simulink model "SimpleVehicle"  (R2018b)
settings: Solver=FixedStepAuto  StartTime=0.0  StopTime=stop_time  FixedStep=global_time_step  RelTol=1e-3
undefined symbols (not defined in the file): car_mass, driver_mass
libraries: nesl_utility x22, fl_lib x12, sdl_lib x5
settings Model: Creator=jbray  LastModifiedBy=Dylan

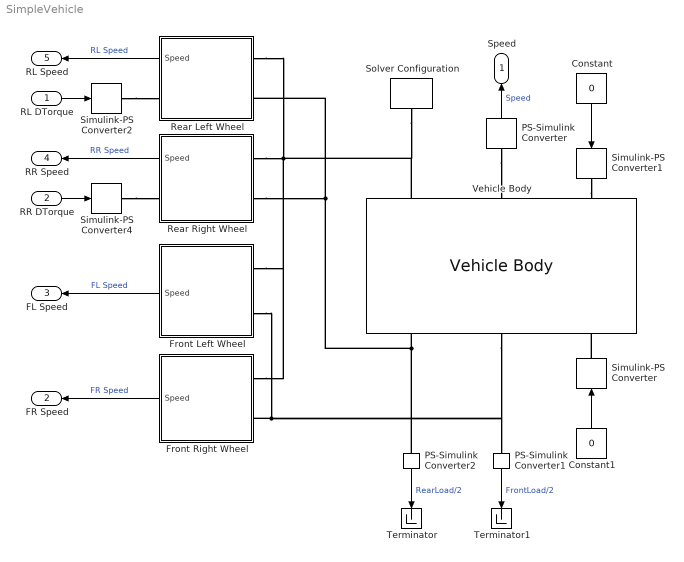
== system SimpleVehicle ==
  RL DTorque : Inport
  RR DTorque : Inport  Port=2
  Constant : Constant  Value=0
  Constant1 : Constant  Value=0
  Front Left Wheel : Subsystem
  Front Right Wheel : Subsystem
  PS-Simulink Converter : nesl_utility/PS-Simulink Converter  PhysicalDomain=network_engine_domain  SubClassName=ps_output  LeftPortType=input  RightPortType=output  PseudoPeriodic=off  Frequencies=[]  Unit=m/s  AffineConversion=off
  PS-Simulink Converter1 : nesl_utility/PS-Simulink Converter  PhysicalDomain=network_engine_domain  SubClassName=ps_output  LeftPortType=input  RightPortType=output  PseudoPeriodic=off  Frequencies=[]  Unit=N  AffineConversion=off
  PS-Simulink Converter2 : nesl_utility/PS-Simulink Converter  PhysicalDomain=network_engine_domain  SubClassName=ps_output  LeftPortType=input  RightPortType=output  PseudoPeriodic=off  Frequencies=[]  Unit=N  AffineConversion=off
  Rear Left Wheel : Subsystem
  Rear Right Wheel : Subsystem
  Simulink-PS Converter : nesl_utility/Simulink-PS Converter  PhysicalDomain=network_engine_domain  SubClassName=ps_input  LeftPortType=input  RightPortType=output  PseudoPeriodic=off  Frequencies=[]  NoiseDistribution=none  NoiseParameters=[]  Unit=rad  AffineConversion=off  FilteringAndDerivatives=provide  SimscapeFilterOrder=1  InputFilterTimeConstant=0.001  UdotUserProvided=0
  Simulink-PS Converter1 : nesl_utility/Simulink-PS Converter  PhysicalDomain=network_engine_domain  SubClassName=ps_input  LeftPortType=input  RightPortType=output  PseudoPeriodic=off  Frequencies=[]  NoiseDistribution=none  NoiseParameters=[]  Unit=m/s  AffineConversion=off  FilteringAndDerivatives=provide  SimscapeFilterOrder=1  InputFilterTimeConstant=0.001  UdotUserProvided=0
  Simulink-PS Converter2 : nesl_utility/Simulink-PS Converter  PhysicalDomain=network_engine_domain  SubClassName=ps_input  LeftPortType=input  RightPortType=output  PseudoPeriodic=off  Frequencies=[]  NoiseDistribution=none  NoiseParameters=[]  Unit=N*m  AffineConversion=off  FilteringAndDerivatives=provide  SimscapeFilterOrder=1  InputFilterTimeConstant=0.001  UdotUserProvided=0
  Simulink-PS Converter4 : nesl_utility/Simulink-PS Converter  PhysicalDomain=network_engine_domain  SubClassName=ps_input  LeftPortType=input  RightPortType=output  PseudoPeriodic=off  Frequencies=[]  NoiseDistribution=none  NoiseParameters=[]  Unit=N*m  AffineConversion=off  FilteringAndDerivatives=provide  SimscapeFilterOrder=1  InputFilterTimeConstant=0.001  UdotUserProvided=0
  Solver Configuration : nesl_utility/Solver Configuration  PhysicalDomain=network_engine_domain  SubClassName=solver  LeftPortType=input  RightPortType=generic  Tones=[]  Harmonics=[]  SimulateNoise=off  Profile=off  UseLocalSampling=off  EnableSwitchedLinearOptims=on  FrequencyDomain=off  UseCCode=off  RelTol=0.001  AbsTol=1e-06  MinStep=1e-09  ToWorkspace=off  RevertToSquareIcSolve=off  NumHomotopyIterations=100  PhasorMode=off  PhasorModeNumHarmonics=1  DoDC=off  ResidualTolerance=1e-09  UseLocalSolver=off  LocalSolverChoice=NE_BACKWARD_EULER_ADVANCER  LocalSolverSampleTime=0.001  DoFixedCost=off  MaxNonlinIter=3  MaxModeIter=2  LinearAlgebra=Sparse  EquationFormulation=NE_TIME_EF  DelaysMemoryBudget=1024  AutomaticFiltering=on  FilteringTimeConstant=0.001  PartitionStorageMethod=AS_NEEDED  PartitionMemoryBudget=1024
  Terminator : Terminator
  Terminator1 : Terminator
  Vehicle Body : sdl_lib/Tires & Vehicles/Vehicle Body  mass=car_mass+driver_mass kg  n_w=2  x_f=CG_front m  x_r=CG_rear m  y_c=CG_height m  model_pitch=1  inertia=pitch_moment_of_inertia kg*m^2  suspension_model=1  k_f=front_suspension_stiffness N/m  b_f=front_suspension_damping N/(m/s)  k_r=rear_suspension_stiffness N/m  b_r=rear_suspension_damping N/(m/s)  k_f_TLU=[-2000, -1000, 0, 1000, 2000] N  x_f_TLU=[-.4, -.2, 0, .2, .4] m  b_f_TLU=[-200, -100, 0, 100, 200] N  v_f_TLU=[-4, -2, 0, 2, 4] m/s  k_r_TLU=[-2000, -1000, 0, 1000, 2000] N  x_r_TLU=[-.4, -.2, 0, .2, .4] m  b_r_TLU=[-200, -100, 0, 100, 200] N  v_r_TLU=[-4, -2, 0, 2, 4] m/s  interp_method=simscape.enum.interpolation.linear  extrap_method=simscape.enum.extrapolation.linear  model_hardstop=0  upper_bound_f=.25 m  lower_bound_f=-.25 m  stop_k_f=1e6 N/m  stop_b_f=150 N/(m/s)  upper_bound_r=.25 m  lower_bound_r=-.25 m  stop_k_r=1e6 N/m  stop_b_r=150 N/(m/s)  initial_pitch=0 rad  initial_pitch_rate=0 rad/s  g=9.81 m/s^2  liftoff_warning=0  area=frontal_area m^2  Cd=drag_coeff  rho=air_density kg/m^3  v_specify=off  v_priority=High  v=0 m/s  v_nominal_specify=off  v_nominal_unit=m/s  v_nominal_value=1
      settings: SourceProductName=Simscape Driveline
  Speed : Outport
  FR Speed : Outport  Port=2
  FL Speed : Outport  Port=3
  RR Speed : Outport  Port=4
  RL Speed : Outport  Port=5
  wires:
  Constant/1 -> Simulink-PS Converter1/1
  RL DTorque/1 -> Simulink-PS Converter2/1
  PS-Simulink Converter/1 -> Speed/1  "Speed"
  PS-Simulink Converter1/1 -> Terminator1/1  "FrontLoad/2"
  PS-Simulink Converter2/1 -> Terminator/1  "RearLoad/2"
  Constant1/1 -> Simulink-PS Converter/1
  Front Right Wheel/1(Speed) -> FR Speed/1  "FR Speed"
  Front Left Wheel/1(Speed) -> FL Speed/1  "FL Speed"
  RR DTorque/1 -> Simulink-PS Converter4/1
  Rear Left Wheel/1(Speed) -> RL Speed/1  "RL Speed"
  Rear Right Wheel/1(Speed) -> RR Speed/1  "RR Speed"
  connections:
  Front Left Wheel/LConn2 -- Vehicle Body/RConn2 -- PS-Simulink Converter1/LConn1 -- Front Right Wheel/LConn2
  Vehicle Body/RConn1 -- PS-Simulink Converter2/LConn1 -- Rear Right Wheel/LConn2 -- Rear Left Wheel/LConn2
  Rear Right Wheel/LConn1 -- Front Left Wheel/LConn1 -- Front Right Wheel/LConn1 -- Rear Left Wheel/LConn1 -- Vehicle Body/LConn1 -- Solver Configuration/RConn1
  Simulink-PS Converter4/RConn1 -- Rear Right Wheel/RConn1
  Simulink-PS Converter2/RConn1 -- Rear Left Wheel/RConn1
  Simulink-PS Converter/RConn1 -- Vehicle Body/RConn3
  PS-Simulink Converter/LConn1 -- Vehicle Body/LConn2
  Simulink-PS Converter1/RConn1 -- Vehicle Body/LConn3

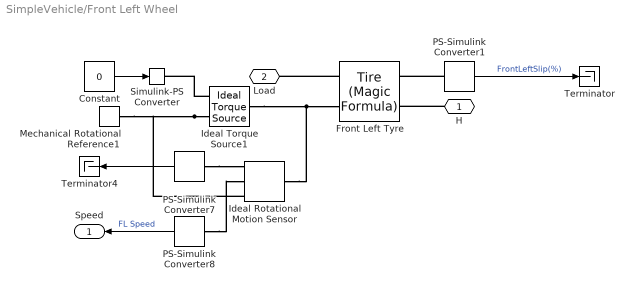
== system SimpleVehicle/Front Left Wheel ==
  Constant : Constant  Value=0
  Front Left Tyre : sdl_lib/Tires & Vehicles/Tire (Magic Formula)  parameterization=2  F_z1=3000 N  F_x1=3500 N  kappa1=10  B_m=magic_B  C_m=magic_C  D_m=magic_D  E_m=magic_E  fz0=4000 N  p_Cx=1.685  p_Dx=[1.21, -.037]  p_Ex=[.344, .095, -.02, 0]  p_Kx=[21.51, -.163, .245]  p_Hx=[-.002, .002]  p_Vx=[0, 0]  v_tr_thr=0.1 m/s  r_e=tyre_radius m  model_compliance=1  stiffness=tyre_stiffness N/m  damping=tyre_damping N/(m/s)  model_inertia=1  inertia=tyre_inertia kg*m^2  initial_velocity=0 rad/s  model_resistance=0  resistance_model=1  coeff=0.015  p_tire=250e3 Pa  alpha=-0.003  beta=0.97  coeff_a=84e-4  coeff_b=6.2e-4 s/m  coeff_c=1.6e-4 s^2/m^2  v_thr=0.001 m/s
      settings: SourceProductName=Simscape Driveline
  Ideal Rotational Motion Sensor : fl_lib/Mechanical/Mechanical Sensors/Ideal Rotational Motion Sensor  offset=0 rad
  Ideal Torque Source1 : fl_lib/Mechanical/Mechanical Sources/Ideal Torque Source
  Mechanical Rotational Reference1 : fl_lib/Mechanical/Rotational Elements/Mechanical Rotational Reference
  PS-Simulink Converter1 : nesl_utility/PS-Simulink Converter  PhysicalDomain=network_engine_domain  SubClassName=ps_output  LeftPortType=input  RightPortType=output  PseudoPeriodic=off  Frequencies=[]  Unit=1  AffineConversion=off
  PS-Simulink Converter7 : nesl_utility/PS-Simulink Converter  PhysicalDomain=network_engine_domain  SubClassName=ps_output  LeftPortType=input  RightPortType=output  PseudoPeriodic=off  Frequencies=[]  Unit=rad  AffineConversion=off
  PS-Simulink Converter8 : nesl_utility/PS-Simulink Converter  PhysicalDomain=network_engine_domain  SubClassName=ps_output  LeftPortType=input  RightPortType=output  PseudoPeriodic=off  Frequencies=[]  Unit=rad/s  AffineConversion=off
  Simulink-PS Converter : nesl_utility/Simulink-PS Converter  PhysicalDomain=network_engine_domain  SubClassName=ps_input  LeftPortType=input  RightPortType=output  PseudoPeriodic=off  Frequencies=[]  NoiseDistribution=none  NoiseParameters=[]  Unit=1  AffineConversion=off  FilteringAndDerivatives=provide  SimscapeFilterOrder=1  InputFilterTimeConstant=0.001  UdotUserProvided=0
  Terminator : Terminator
  Terminator4 : Terminator
  H : PMIOPort  Side=Left
  Load : PMIOPort  Port=2  Side=Left
  Speed : Outport
  wires:
  PS-Simulink Converter1/1 -> Terminator/1  "FrontLeftSlip(%)"
  PS-Simulink Converter8/1 -> Speed/1  "FL Speed"
  PS-Simulink Converter7/1 -> Terminator4/1
  Constant/1 -> Simulink-PS Converter/1
  connections:
  Front Left Tyre/LConn1 -- Load/RConn1
  PS-Simulink Converter1/LConn1 -- Front Left Tyre/RConn1
  H/RConn1 -- Front Left Tyre/RConn2
  PS-Simulink Converter7/LConn1 -- Ideal Rotational Motion Sensor/RConn3
  PS-Simulink Converter8/LConn1 -- Ideal Rotational Motion Sensor/RConn2
  Ideal Torque Source1/RConn1 -- Simulink-PS Converter/RConn1
  Ideal Rotational Motion Sensor/LConn1 -- Ideal Torque Source1/LConn1 -- Front Left Tyre/LConn2
  Ideal Torque Source1/RConn2 -- Ideal Rotational Motion Sensor/RConn1 -- Mechanical Rotational Reference1/LConn1

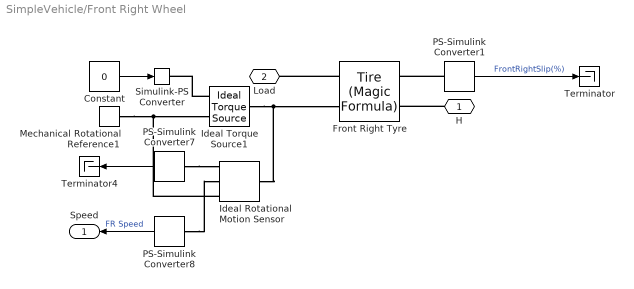
== system SimpleVehicle/Front Right Wheel ==
  Constant : Constant  Value=0
  Front Right Tyre : sdl_lib/Tires & Vehicles/Tire (Magic Formula)  parameterization=2  F_z1=3000 N  F_x1=3500 N  kappa1=10  B_m=magic_B  C_m=magic_C  D_m=magic_D  E_m=magic_E  fz0=4000 N  p_Cx=1.685  p_Dx=[1.21, -.037]  p_Ex=[.344, .095, -.02, 0]  p_Kx=[21.51, -.163, .245]  p_Hx=[-.002, .002]  p_Vx=[0, 0]  v_tr_thr=0.1 m/s  r_e=tyre_radius m  model_compliance=1  stiffness=tyre_stiffness N/m  damping=tyre_damping N/(m/s)  model_inertia=1  inertia=tyre_inertia kg*m^2  initial_velocity=0 rad/s  model_resistance=0  resistance_model=1  coeff=0.015  p_tire=250e3 Pa  alpha=-0.003  beta=0.97  coeff_a=84e-4  coeff_b=6.2e-4 s/m  coeff_c=1.6e-4 s^2/m^2  v_thr=0.001 m/s
      settings: SourceProductName=Simscape Driveline
  Ideal Rotational Motion Sensor : fl_lib/Mechanical/Mechanical Sensors/Ideal Rotational Motion Sensor  offset=0 rad
  Ideal Torque Source1 : fl_lib/Mechanical/Mechanical Sources/Ideal Torque Source
  Mechanical Rotational Reference1 : fl_lib/Mechanical/Rotational Elements/Mechanical Rotational Reference
  PS-Simulink Converter1 : nesl_utility/PS-Simulink Converter  PhysicalDomain=network_engine_domain  SubClassName=ps_output  LeftPortType=input  RightPortType=output  PseudoPeriodic=off  Frequencies=[]  Unit=1  AffineConversion=off
  PS-Simulink Converter7 : nesl_utility/PS-Simulink Converter  PhysicalDomain=network_engine_domain  SubClassName=ps_output  LeftPortType=input  RightPortType=output  PseudoPeriodic=off  Frequencies=[]  Unit=rad  AffineConversion=off
  PS-Simulink Converter8 : nesl_utility/PS-Simulink Converter  PhysicalDomain=network_engine_domain  SubClassName=ps_output  LeftPortType=input  RightPortType=output  PseudoPeriodic=off  Frequencies=[]  Unit=rad/s  AffineConversion=off
  Simulink-PS Converter : nesl_utility/Simulink-PS Converter  PhysicalDomain=network_engine_domain  SubClassName=ps_input  LeftPortType=input  RightPortType=output  PseudoPeriodic=off  Frequencies=[]  NoiseDistribution=none  NoiseParameters=[]  Unit=1  AffineConversion=off  FilteringAndDerivatives=provide  SimscapeFilterOrder=1  InputFilterTimeConstant=0.001  UdotUserProvided=0
  Terminator : Terminator
  Terminator4 : Terminator
  H : PMIOPort  Side=Left
  Load : PMIOPort  Port=2  Side=Left
  Speed : Outport
  wires:
  PS-Simulink Converter7/1 -> Terminator4/1
  PS-Simulink Converter8/1 -> Speed/1  "FR Speed"
  PS-Simulink Converter1/1 -> Terminator/1  "FrontRightSlip(%)"
  Constant/1 -> Simulink-PS Converter/1
  connections:
  Mechanical Rotational Reference1/LConn1 -- Ideal Torque Source1/RConn2 -- Ideal Rotational Motion Sensor/RConn1
  Ideal Torque Source1/LConn1 -- Front Right Tyre/LConn2 -- Ideal Rotational Motion Sensor/LConn1
  Ideal Torque Source1/RConn1 -- Simulink-PS Converter/RConn1
  PS-Simulink Converter8/LConn1 -- Ideal Rotational Motion Sensor/RConn2
  PS-Simulink Converter7/LConn1 -- Ideal Rotational Motion Sensor/RConn3
  H/RConn1 -- Front Right Tyre/RConn2
  PS-Simulink Converter1/LConn1 -- Front Right Tyre/RConn1
  Front Right Tyre/LConn1 -- Load/RConn1

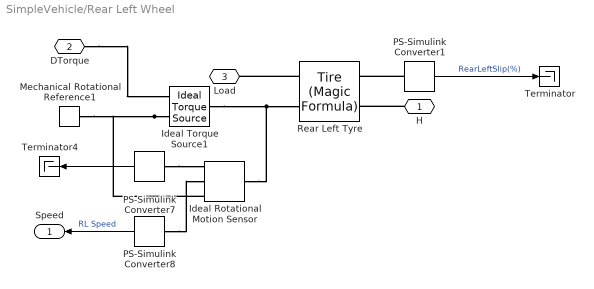
== system SimpleVehicle/Rear Left Wheel ==
  Ideal Rotational Motion Sensor : fl_lib/Mechanical/Mechanical Sensors/Ideal Rotational Motion Sensor  offset=0 rad
  Ideal Torque Source1 : fl_lib/Mechanical/Mechanical Sources/Ideal Torque Source
  Mechanical Rotational Reference1 : fl_lib/Mechanical/Rotational Elements/Mechanical Rotational Reference
  PS-Simulink Converter1 : nesl_utility/PS-Simulink Converter  PhysicalDomain=network_engine_domain  SubClassName=ps_output  LeftPortType=input  RightPortType=output  PseudoPeriodic=off  Frequencies=[]  Unit=1  AffineConversion=off
  PS-Simulink Converter7 : nesl_utility/PS-Simulink Converter  PhysicalDomain=network_engine_domain  SubClassName=ps_output  LeftPortType=input  RightPortType=output  PseudoPeriodic=off  Frequencies=[]  Unit=rad  AffineConversion=off
  PS-Simulink Converter8 : nesl_utility/PS-Simulink Converter  PhysicalDomain=network_engine_domain  SubClassName=ps_output  LeftPortType=input  RightPortType=output  PseudoPeriodic=off  Frequencies=[]  Unit=rad/s  AffineConversion=off
  Rear Left Tyre : sdl_lib/Tires & Vehicles/Tire (Magic Formula)  parameterization=2  F_z1=3000 N  F_x1=3500 N  kappa1=10  B_m=magic_B  C_m=magic_C  D_m=magic_D  E_m=magic_E  fz0=4000 N  p_Cx=1.685  p_Dx=[1.21, -.037]  p_Ex=[.344, .095, -.02, 0]  p_Kx=[21.51, -.163, .245]  p_Hx=[-.002, .002]  p_Vx=[0, 0]  v_tr_thr=0.1 m/s  r_e=tyre_radius m  model_compliance=1  stiffness=tyre_stiffness N/m  damping=tyre_damping N/(m/s)  model_inertia=1  inertia=tyre_inertia kg*m^2  initial_velocity=0 rad/s  model_resistance=0  resistance_model=1  coeff=0.015  p_tire=250e3 Pa  alpha=-0.003  beta=0.97  coeff_a=84e-4  coeff_b=6.2e-4 s/m  coeff_c=1.6e-4 s^2/m^2  v_thr=0.001 m/s
      settings: SourceProductName=Simscape Driveline
  Terminator : Terminator
  Terminator4 : Terminator
  H : PMIOPort  Side=Left
  DTorque : PMIOPort  Port=2  Side=Right
  Load : PMIOPort  Port=3  Side=Left
  Speed : Outport
  wires:
  PS-Simulink Converter1/1 -> Terminator/1  "RearLeftSlip(%)"
  PS-Simulink Converter8/1 -> Speed/1  "RL Speed"
  PS-Simulink Converter7/1 -> Terminator4/1
  connections:
  Rear Left Tyre/LConn1 -- Load/RConn1
  PS-Simulink Converter1/LConn1 -- Rear Left Tyre/RConn1
  H/RConn1 -- Rear Left Tyre/RConn2
  PS-Simulink Converter7/LConn1 -- Ideal Rotational Motion Sensor/RConn3
  PS-Simulink Converter8/LConn1 -- Ideal Rotational Motion Sensor/RConn2
  DTorque/RConn1 -- Ideal Torque Source1/RConn1
  Ideal Rotational Motion Sensor/LConn1 -- Ideal Torque Source1/LConn1 -- Rear Left Tyre/LConn2
  Ideal Torque Source1/RConn2 -- Ideal Rotational Motion Sensor/RConn1 -- Mechanical Rotational Reference1/LConn1

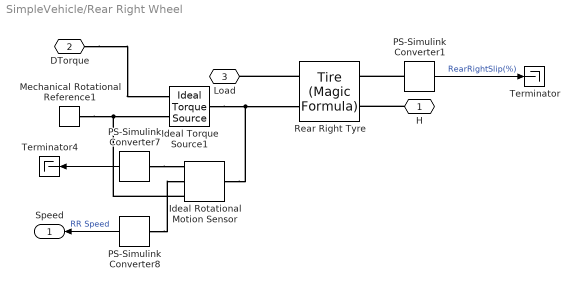
== system SimpleVehicle/Rear Right Wheel ==
  Ideal Rotational Motion Sensor : fl_lib/Mechanical/Mechanical Sensors/Ideal Rotational Motion Sensor  offset=0 rad
  Ideal Torque Source1 : fl_lib/Mechanical/Mechanical Sources/Ideal Torque Source
  Mechanical Rotational Reference1 : fl_lib/Mechanical/Rotational Elements/Mechanical Rotational Reference
  PS-Simulink Converter1 : nesl_utility/PS-Simulink Converter  PhysicalDomain=network_engine_domain  SubClassName=ps_output  LeftPortType=input  RightPortType=output  PseudoPeriodic=off  Frequencies=[]  Unit=1  AffineConversion=off
  PS-Simulink Converter7 : nesl_utility/PS-Simulink Converter  PhysicalDomain=network_engine_domain  SubClassName=ps_output  LeftPortType=input  RightPortType=output  PseudoPeriodic=off  Frequencies=[]  Unit=rad  AffineConversion=off
  PS-Simulink Converter8 : nesl_utility/PS-Simulink Converter  PhysicalDomain=network_engine_domain  SubClassName=ps_output  LeftPortType=input  RightPortType=output  PseudoPeriodic=off  Frequencies=[]  Unit=rad/s  AffineConversion=off
  Rear Right Tyre : sdl_lib/Tires & Vehicles/Tire (Magic Formula)  parameterization=2  F_z1=3000 N  F_x1=3500 N  kappa1=10  B_m=magic_B  C_m=magic_C  D_m=magic_D  E_m=magic_E  fz0=4000 N  p_Cx=1.685  p_Dx=[1.21, -.037]  p_Ex=[.344, .095, -.02, 0]  p_Kx=[21.51, -.163, .245]  p_Hx=[-.002, .002]  p_Vx=[0, 0]  v_tr_thr=0.1 m/s  r_e=tyre_radius m  model_compliance=1  stiffness=tyre_stiffness N/m  damping=tyre_damping N/(m/s)  model_inertia=1  inertia=tyre_inertia kg*m^2  initial_velocity=0 rad/s  model_resistance=0  resistance_model=1  coeff=0.015  p_tire=250e3 Pa  alpha=-0.003  beta=0.97  coeff_a=84e-4  coeff_b=6.2e-4 s/m  coeff_c=1.6e-4 s^2/m^2  v_thr=0.001 m/s
      settings: SourceProductName=Simscape Driveline
  Terminator : Terminator
  Terminator4 : Terminator
  H : PMIOPort  Side=Left
  DTorque : PMIOPort  Port=2  Side=Right
  Load : PMIOPort  Port=3  Side=Left
  Speed : Outport
  wires:
  PS-Simulink Converter7/1 -> Terminator4/1
  PS-Simulink Converter8/1 -> Speed/1  "RR Speed"
  PS-Simulink Converter1/1 -> Terminator/1  "RearRightSlip(%)"
  connections:
  Mechanical Rotational Reference1/LConn1 -- Ideal Rotational Motion Sensor/RConn1 -- Ideal Torque Source1/RConn2
  Ideal Torque Source1/LConn1 -- Rear Right Tyre/LConn2 -- Ideal Rotational Motion Sensor/LConn1
  DTorque/RConn1 -- Ideal Torque Source1/RConn1
  PS-Simulink Converter8/LConn1 -- Ideal Rotational Motion Sensor/RConn2
  PS-Simulink Converter7/LConn1 -- Ideal Rotational Motion Sensor/RConn3
  H/RConn1 -- Rear Right Tyre/RConn2
  PS-Simulink Converter1/LConn1 -- Rear Right Tyre/RConn1
  Rear Right Tyre/LConn1 -- Load/RConn1
